simulink model "GestuerteGerichter"  (R2023b)
settings: Solver=ode23tb  StartTime=0.0  StopTime=0.1  FixedStep=1e-5  MaxStep=1e-4  RelTol=1e-3
InitFcn:
  | % Power source (Voltage of Volts RMS Pha-Pha)
  | v_ac = 100;
  | % frequency of AC
  | f_ac = 50;
  | % Resistor of Motor
  | R_GM = 1;
  | % Inductance of Motor
  | L_GM = 20e-3;
undefined symbols (not defined in the file): D1, lagging, pulse
libraries: spsMultimeterLib x3, spsDCVoltageSourceLib x1, spsGroundLib x1, spsCurrentMeasurementLib x1, spsMeanLib x1, spsPLL3phLib x1, spsPulseGeneratorThyristor6PulseLib x1, simulink_extras x1, spsSeriesRLCBranchLib x1, spsThreePhaseProgrammableVoltageSourceLib x1, spsThreePhaseVIMeasurementLib x1, spsUniversalBridgeLib x1
settings Model: Creator=email  LastModifiedBy=email
settings SolverCC: SolverResetMethod=Robust

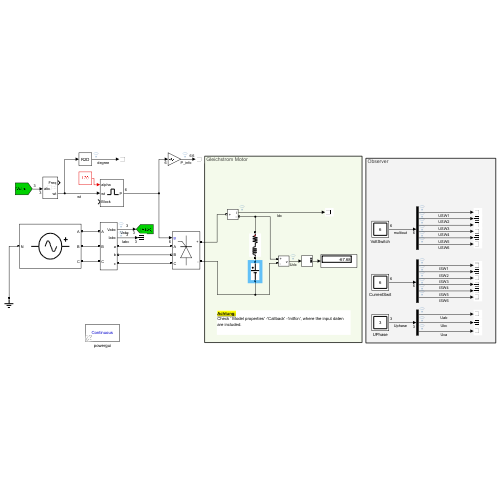
[thumbnail: Simulink's stored preview of the top-level diagram]
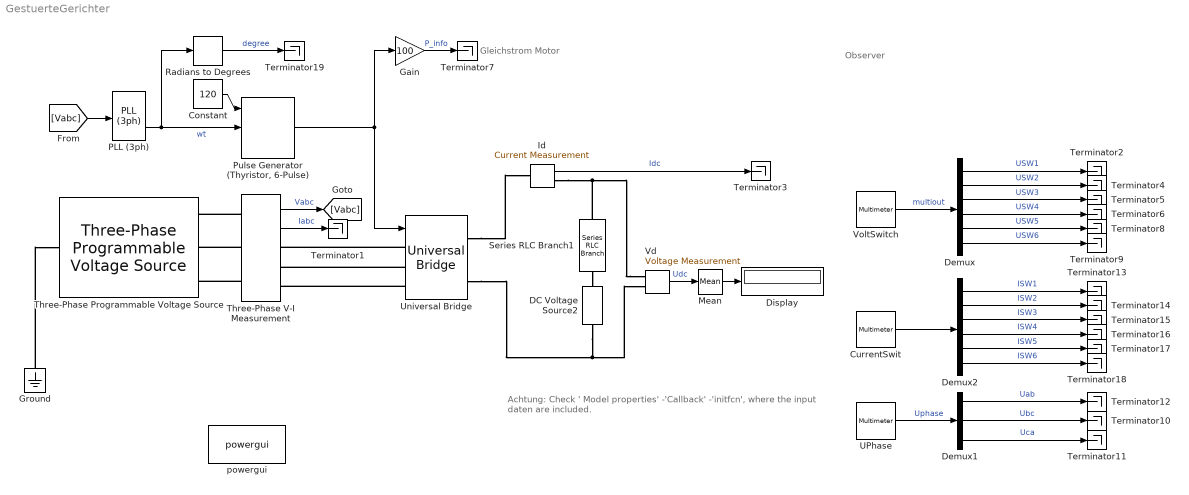
== system GestuerteGerichter ==
  note: Achtung:
      | Check ' Model properties' -'Callback' -'initfcn', where the input daten are included.
  note: Observer
  note: Gleichstrom Motor
  Constant : Constant  Value=120
  CurrentSwit : spsMultimeterLib/Multimeter  L=16  sel=[11 12 13 14 15 16]  yselected={}  Gain=[1 1 1 1 1 1]  OutputType=Complex  PlotAtSimulationStop=off  PhasorSimulation=off
  DC Voltage Source2 : spsDCVoltageSourceLib/DC Voltage Source  Description=source block  Amplitude=-150  Measurements=None
      settings: AttributesFormatString=\n
  Demux : Demux  Outputs=6
  Demux1 : Demux  Outputs=3
  Demux2 : Demux  Outputs=6
  Display : Display
  Gain : Gain  Gain=100
  Ground : spsGroundLib/Ground  LConnTagsString=a
  Id : spsCurrentMeasurementLib/Current Measurement  Tag=PoWeRsYsTeMmEaSuReMeNt  PhasorSimulation=off  OutputType=Complex  PSBequivalent=0
      settings: AttributesFormatString=\n
  Mean : spsMeanLib/Mean  Freq=f_ac  Vinit=0  Ts=0
  PLL (3ph) : spsPLL3phLib/PLL (3ph)  Fmin=1  Par_Init=[0, f_ac]  ParK=[180, 3200, 1]  TcD=1e-4  MaxRateChangeFreq=12  FilterCutOffFreq=25  Ts=0  AGC=on
  "Pulse Generator (Thyristor, 6-Pulse)" : spsPulseGeneratorThyristor6PulseLib/Pulse Generator (Thyristor, 6-Pulse)  GenType=6-pulse  Delta=D1 (lagging)  pwidth=10  Double_Pulse=off  Ts=0
      settings: LibrarySourceBlock=|
      | sps_lib/Power Electronics/Power Electronics Control/Pulse Generator
      | (Thyristor, 6-Pulse)
  Radians to Degrees : simulink_extras/Transformations/Radians to Degrees
  Series RLC Branch1 : spsSeriesRLCBranchLib/Series RLC Branch  LConnTagsString=__new0  RConnTagsString=__new0  BranchType=RL  Resistance=R_GM  Inductance=L_GM  SetiL0=off  InitialCurrent=0.1  Capacitance=inf  Setx0=off  InitialVoltage=0  Measurements=None
  Terminator{1..19} (19 alike) : Terminator
  Three-Phase Programmable Voltage Source : spsThreePhaseProgrammableVoltageSourceLib/Three-Phase Programmable Voltage Source  PositiveSequence="[v_ac  0 f_ac]"  VariationEntity=None  VariationType=Table of time-amplitude pairs  VariationTypeAlt=Step  VariationStep=0.5  VariationRate=10  VariationMagnitude=0.3  VariationFrequency=2  VariationTiming=[1 2]  VariationPhaseA=off  Amplitudes=[1 0.8 1.2 1.0]  TimeValues=[0 0.1 0.15 0.2]  HarmonicGeneration=off  HarmonicA=[3 0.2 -25 0]  HarmonicB=[2 0.15 35 2]  Timing="[0.05  3]"  BusType=swing  Pref=0  Qref=0  Qmin=-inf  Qmax=inf
  Three-Phase V-I Measurement : spsThreePhaseVIMeasurementLib/Three-Phase V-I Measurement  VoltageMeasurement=phase-to-ground  SetLabelV=off  LabelV=Vabc  Vpu=off  VpuLL=off  CurrentMeasurement=yes  SetLabelI=off  LabelI=Iabc  Ipu=off  Pbase=100e6  Vbase=500e3  OutputType=Complex  PhasorSimulation=off  PSBequivalent=0
  UPhase : spsMultimeterLib/Multimeter  L=16  sel=[7 8 9]  yselected={}  Gain=[1 1 1]  OutputType=Complex  PlotAtSimulationStop=off  PhasorSimulation=off
  Universal Bridge : spsUniversalBridgeLib/Universal Bridge  Arms=3  SnubberResistance=1e5  SnubberCapacitance=inf  Device=Thyristors  Ron=1e-3  Lon=0  ForwardVoltages="[  0  0  ]"  ForwardVoltage=0  GTOparameters=[ 10e-6 , 20e-6 ]  IGBTparameters=[ 1e-6 , 2e-6 ]  Measurements=All voltages and currents  Measurements_2=None  converterType=Rectifier
  Vd : spsVoltageMeasurementLib/Voltage Measurement  Tag=PoWeRsYsTeMmEaSuReMeNt  PhasorSimulation=off  OutputType=Complex  PSBequivalent=0
  VoltSwitch : spsMultimeterLib/Multimeter  L=16  sel=[1 2 3 4 5 6]  yselected={}  Gain=[1 1 1 1 1 1]  OutputType=Complex  PlotAtSimulationStop=off  PhasorSimulation=off
  powergui : sps_lib/powergui  Priority=1  SimulationMode=Continuous  SampleTime=1e-5  frequency=60  Iterations=50  frequencyindice=50  Pbase=100e6  ErrMax=1e-4  UnitsV=kV  UnitsW=MW  buscounter=0  FunctionMessages=off  echomessages=off  EnableUseOfTLC=off  CurrentSourceSwitches=off  DisableSnubberDevices=off  DisableRonSwitches=off  DisableVfSwitches=off  DisplayEquations=off  AutomaticDiscreteSolvers=off  SolverType=Tustin/Backward Euler (TBE)  Interpol=off  ExternalGateDelay=off  methode=off  Ts=100  x0status=blocks  SPID=on  SwTol=0  HookPort=off  NonlinearTolerance=1e-4  nMaxIteration=100  ContinueOnMaxIteration=off  RestoreLinks=warning  ResistiveCurrentMeasurement=off  Frange=[0:2:500]  Ylog=off  Xlog=on  ShowGrid=off  save=off  variable=ZData  structure=0  ZoomFFT=off  StartTime=0.0  cycles=1  DisplayStyle=1  fundamental=60  FreqAxis=off  MaxFrequency=1000  frequencyindicesteady=1  RmsSteady=1  display=off
  wires:
  Three-Phase V-I Measurement/1 -> [Vabc]  "Vabc"
  PLL (3ph)/2 -> Radians to Degrees/1, "Pulse Generator (Thyristor, 6-Pulse)"/2  "wt"
  Constant/1 -> "Pulse Generator (Thyristor, 6-Pulse)"/1
  Three-Phase V-I Measurement/2 -> Terminator1/1  "Iabc"
  Id/1 -> Terminator3/1  "Idc"
  Vd/1 -> Mean/1  "Udc"
  Mean/1 -> Display/1
  VoltSwitch/1 -> Demux/1  "multiout"
  Demux/1 -> Terminator2/1  "USW1"
  Demux/2 -> Terminator4/1  "USW2"
  Demux/3 -> Terminator5/1  "USW3"
  Demux/4 -> Terminator6/1  "USW4"
  [Vabc] -> PLL (3ph)/1
  Demux/5 -> Terminator8/1  "USW5"
  Demux/6 -> Terminator9/1  "USW6"
  UPhase/1 -> Demux1/1  "Uphase"
  Demux1/1 -> Terminator12/1  "Uab"
  Demux1/2 -> Terminator10/1  "Ubc"
  Demux1/3 -> Terminator11/1  "Uca"
  Demux2/6 -> Terminator18/1  "ISW6"
  Demux2/5 -> Terminator17/1  "ISW5"
  Demux2/1 -> Terminator13/1  "ISW1"
  Demux2/3 -> Terminator15/1  "ISW3"
  Demux2/4 -> Terminator16/1  "ISW4"
  CurrentSwit/1 -> Demux2/1
  Demux2/2 -> Terminator14/1  "ISW2"
  "Pulse Generator (Thyristor, 6-Pulse)"/1 -> Gain/1, Universal Bridge/1
  Gain/1 -> Terminator7/1  "P_info"
  Radians to Degrees/1 -> Terminator19/1  "degree"
  connections:
  Ground/LConn1 -- Three-Phase Programmable Voltage Source/LConn1
  Three-Phase V-I Measurement/LConn2 -- Three-Phase Programmable Voltage Source/RConn2
  Three-Phase V-I Measurement/LConn1 -- Three-Phase Programmable Voltage Source/RConn1
  Three-Phase V-I Measurement/LConn3 -- Three-Phase Programmable Voltage Source/RConn3
  Universal Bridge/LConn3 -- Three-Phase V-I Measurement/RConn3
  Universal Bridge/LConn2 -- Three-Phase V-I Measurement/RConn2
  Universal Bridge/LConn1 -- Three-Phase V-I Measurement/RConn1
  Vd/LConn1 -- Series RLC Branch1/LConn1 -- Id/RConn1
  Universal Bridge/RConn2 -- DC Voltage Source2/LConn1 -- Vd/LConn2
  Universal Bridge/RConn1 -- Id/LConn1
  Series RLC Branch1/RConn1 -- DC Voltage Source2/RConn1
